simulink model "sim_tracking_2"  (R2023b)
settings: Solver=ode45  StartTime=0.0  StopTime=Tfin  FixedStep=3  RelTol=1e-3  EnableMultiTasking=on
values from neighbouring files (symbols this model uses):
  IJ = inv(J)    [main_regulation.m]    (also in main_tracking_1.m; main_tracking_2.m)
  J = diag([10 9 12]*1e3)    [main_regulation.m]    (also in main_tracking_1.m; main_tracking_2.m = diag(J0))
  J0 = [10 9 12]*1e3    [main_tracking_2.m]
  q0 = [0.6853;0.6953;0.1531;0.1531]    [main_regulation.m]    (also in main_tracking_1.m = [cos(th0/2);0;sin(th0/2);0]; main_tracking_2.m = [1;0;0;0]; simulation_dyn_kin.m = [1;0;0;0])
  satu = 150    [main_tracking_2.m]
  w0 = [0.53;0.53;0.053]    [main_regulation.m]    (also in main_tracking_1.m = [0;0;0]; main_tracking_2.m = [0;0;0]; simulation_dyn_kin.m = [0.01;0;1]; simulation_euler.m = [0.25;0;0.63])
  wr = [0;0;0]    [main_tracking_1.m]    (also in main_tracking_2.m = [0.3;0;0])
libraries: vrlib x1
settings Model: Creator=carlonovara  LastModifiedBy=carlonovara
settings SolverCC: AlgebraicLoopSolver=TrustRegion
settings DataIOCC: ReturnWorkspaceOutputs=off
settings OptimizationCC: LifeSpan=inf
settings DebuggingCC: UnconnectedInputMsg=warning  UnconnectedOutputMsg=warning  UnconnectedLineMsg=warning  SFUnexpectedBacktrackingDiag=warning  SFNoUnconditionalDefaultTransitionDiag=warning  SFExecutionAtInitializationDiag=none  ArithmeticOperatorsInVariantConditions=warning
settings ModelReferenceCC: EnableRefExpFcnMdlSchedulingChecks=on
settings SFSimCC: SimUseLocalCustomCode=off  CustomCodeUndefinedFunction=UseInterfaceOnly
settings RTWCC: RTWUseLocalCustomCode=off
settings CodeAppCC: StateflowObjectComments=on
settings GRTTargetCC: TargetLangStandard=C89/C90 (ANSI)
settings ConfigComp: CovMetricSettings=dw  CovSaveCumulativeToWorkspaceVar=on  CovSaveSingleToWorkspaceVar=on  CovExternalEMLEnable=off

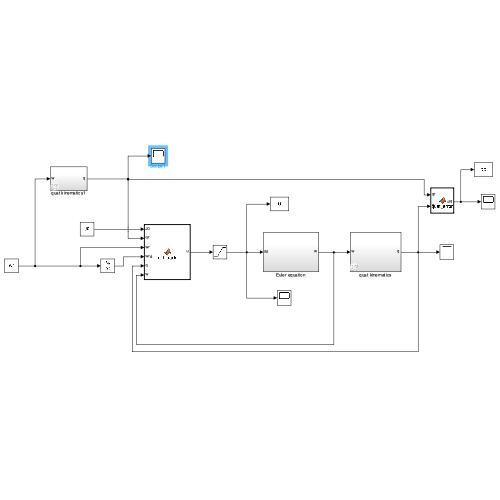
[thumbnail: Simulink's stored preview of the top-level diagram]
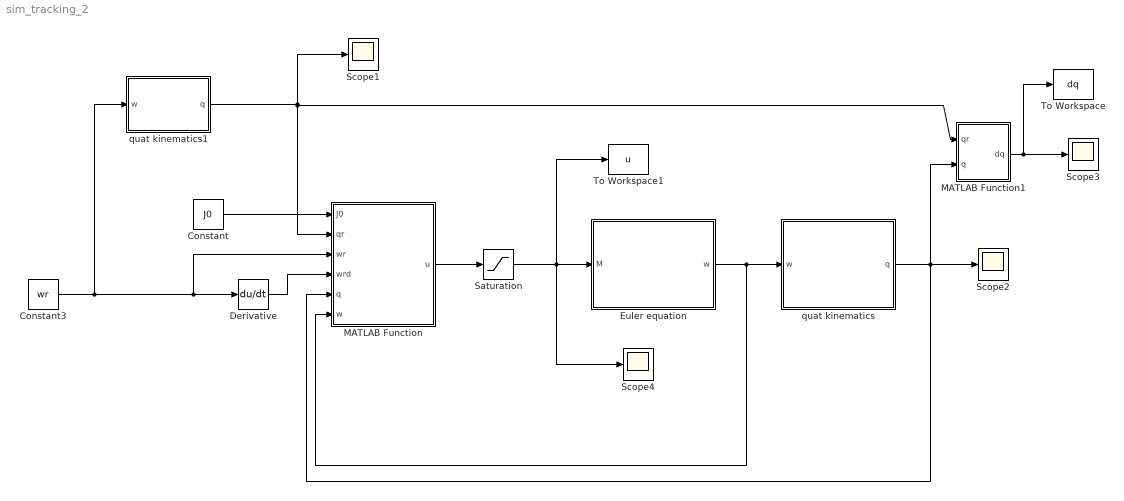
== system sim_tracking_2 ==
  Constant : Constant  Value=J0
  Constant3 : Constant  Value=wr
  Derivative : Derivative  CoefficientInTFapproximation=100
  Euler equation : Subsystem
  MATLAB Function : MATLAB Function  TreatAsAtomicUnit=on
  MATLAB Function1 : MATLAB Function  TreatAsAtomicUnit=on
  Saturation : Saturate  UpperLimit=satu  LowerLimit=-satu
  Scope{1..4} (4 alike) : Scope
  To Workspace : ToWorkspace  VariableName=dq  SaveFormat=Timeseries  SampleTime=-1
  To Workspace1 : ToWorkspace  VariableName=u  SaveFormat=Timeseries  SampleTime=-1
  quat kinematics : Subsystem  AncestorBlock=lib_rotations_2014/quat kinematics
  quat kinematics1 : Subsystem  AncestorBlock=lib_rotations_2014/quat kinematics
  wires:
  MATLAB Function/1(u) -> Saturation/1
  Euler equation/1(w) -> quat kinematics/1(w), MATLAB Function/6(w)
  quat kinematics1/1(q) -> Scope1/1, MATLAB Function1/1(qr), MATLAB Function/2(qr)
  quat kinematics/1(q) -> MATLAB Function1/2(q), MATLAB Function/5(q), Scope2/1
  Constant3/1 -> quat kinematics1/1(w), MATLAB Function/3(wr), Derivative/1
  Derivative/1 -> MATLAB Function/4(wrd)
  MATLAB Function1/1(dq) -> To Workspace/1, Scope3/1
  Constant/1 -> MATLAB Function/1(J0)
  Saturation/1 -> To Workspace1/1, Scope4/1, Euler equation/1(M)

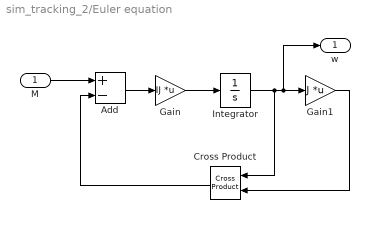
== system sim_tracking_2/Euler equation ==
  M : Inport
  Add : Sum  Inputs=+-
  Cross Product : vrlib/Utilities/Cross Product
  Gain : Gain  Gain=IJ  Multiplication=Matrix(K*u)
  Gain1 : Gain  Gain=J  Multiplication=Matrix(K*u)
  Integrator : Integrator  InitialCondition=w0
  w : Outport  VectorParamsAs1DForOutWhenUnconnected=off
  wires:
  M/1 -> Add/1
  Integrator/1 -> Cross Product/1, w/1, Gain1/1
  Gain/1 -> Integrator/1
  Gain1/1 -> Cross Product/2
  Add/1 -> Gain/1
  Cross Product/1 -> Add/2

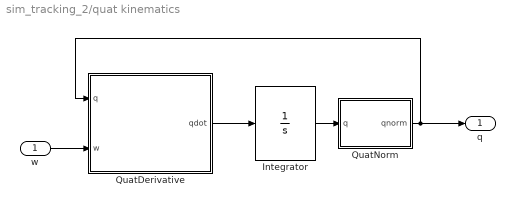
== system sim_tracking_2/quat kinematics ==
  w : Inport  PortDimensions=3
  Integrator : Integrator  InitialCondition=q0
  QuatDerivative : MATLAB Function  TreatAsAtomicUnit=on
  QuatNorm : MATLAB Function  TreatAsAtomicUnit=on
  q : Outport  PortDimensions=4  VectorParamsAs1DForOutWhenUnconnected=off
  wires:
  w/1 -> QuatDerivative/2(w)
  QuatDerivative/1(qdot) -> Integrator/1
  QuatNorm/1(qnorm) -> QuatDerivative/1(q), q/1
  Integrator/1 -> QuatNorm/1(q)

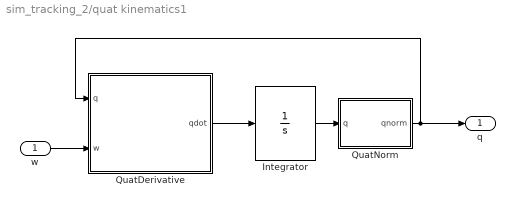
== system sim_tracking_2/quat kinematics1 ==
  w : Inport  PortDimensions=3
  Integrator : Integrator  InitialCondition=[1;0;0;0]
  QuatDerivative : MATLAB Function  TreatAsAtomicUnit=on
  QuatNorm : MATLAB Function  TreatAsAtomicUnit=on
  q : Outport  PortDimensions=4  VectorParamsAs1DForOutWhenUnconnected=off
  wires:
  Integrator/1 -> QuatNorm/1(q)
  QuatNorm/1(qnorm) -> q/1, QuatDerivative/1(q)
  QuatDerivative/1(qdot) -> Integrator/1
  w/1 -> QuatDerivative/2(w)

== matlab function sim_tracking_2/quat kinematics/QuatDerivative ==
  data: q input; qdot output; w input
function qdot= QuatDerivative(q,w)
%#codegen
omegaq=[0; w];
Q=[q(1) -q(2) -q(3) -q(4);
    q(2) q(1) -q(4) q(3);
    q(3) q(4) q(1) -q(2);
    q(4) -q(3) q(2) q(1)];
qdot=Q*omegaq/2;

== matlab function sim_tracking_2/MATLAB Function ==
  data: J0 input; qr input; wr input; wrd input; q input; u output; w input
function u = ctrl_track(J0,qr,wr,wrd,q,w)
%#codegen

J=diag(J0);

u=zeros(3,1);

qs=[q(1);-q(2:4)];
dq=quatprod(qs,qr);
dw=wr-w;

% Proportional-Derivative controller
% kp=2;
% kd=200;
% u=kp*dq(2:4)+kd*dw;
% %u=kp*sign(dq(1))*dq(2:4)+kd*dw;

% Sliding Mode Control - version 1
k2=1;
k1=100;
eta=200;
us=J*(wrd+k2/2*(dq(1)*dw+crossprod(dq(2:4),wr+w)))+crossprod(w,J*w);
s=dw+k2*dq(2:4);
u=us+k1*tanh(eta*s);

% Sliding Mode Control - version 2
% k2=0.1;
% k1=50;
% us=J*(wrd+k2/2*(abs(dq(1))*dw+sign(q(1))*crossprod(dq(2:4),wr+w)))+crossprod(w,J*w);
% s=dw+k2*sign(q(1))*dq(2:4);
% u=us+k1*tanh(s);

end

== matlab function sim_tracking_2/quat kinematics/QuatNorm ==
  data: q input; qnorm output
function qnorm = QuatNorm(q)
%#codegen
qnorm=zeros(4,1);
q2=sqrt(q'*q);
qnorm=q/q2;

== matlab function sim_tracking_2/quat kinematics1/QuatDerivative ==
  data: q input; qdot output; w input
function qdot= QuatDerivative(q,w)
%#codegen
omegaq=[0; w];
Q=[q(1) -q(2) -q(3) -q(4);
    q(2) q(1) -q(4) q(3);
    q(3) q(4) q(1) -q(2);
    q(4) -q(3) q(2) q(1)];
qdot=Q*omegaq/2;

== matlab function sim_tracking_2/quat kinematics1/QuatNorm ==
  data: q input; qnorm output
function qnorm = QuatNorm(q)
%#codegen
qnorm=zeros(4,1);
q2=sqrt(q'*q);
qnorm=q/q2;

== matlab function sim_tracking_2/MATLAB Function1 ==
  data: qr input; q input; dq output
function dq = quat_error(qr,q)
%#codegen

qs=[q(1);-q(2:4)];
dq=quatprod(qs,qr);

end
